simulink subsystem "eulerAngles2Quat"  (R2026a)
settings: Solver=VariableStepAuto
values from neighbouring files (symbols this model uses):
  navControl = 1    [navParams.sldd]
libraries: aerolibutil x1, sharedutil x1
settings Model: Creator=maxhu  LastModifiedBy=maxhu

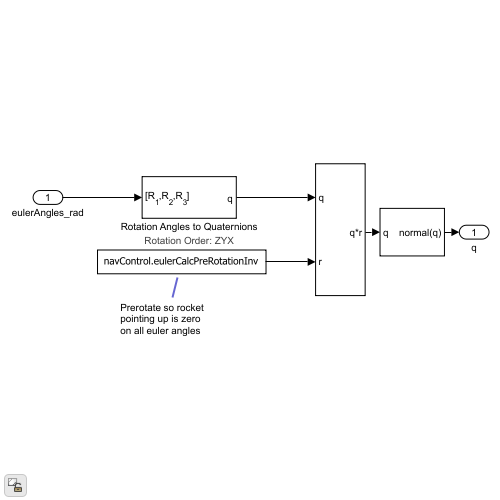
[thumbnail: Simulink's stored preview of the top-level diagram]
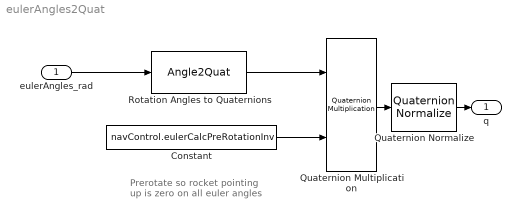
== system eulerAngles2Quat ==
  note: Prerotate so rocket pointing up is zero on all euler angles
  eulerAngles_rad : Inport
  Constant : Constant  Value=navControl.eulerCalcPreRotationInv
  Quaternion Multiplication : aerolibutil/Quaternion Multiplication
  Quaternion Normalize : sharedutil/Quaternion Normalize  aMode=aMode
  Rotation Angles to Quaternions : Angle2Quat
      settings: AttributesFormatString=Rotation Order: %<rotationOrder>
  q : Outport
  wires:
  Constant/1 -> Quaternion Multiplication/2
  eulerAngles_rad/1 -> Rotation Angles to Quaternions/1
  Rotation Angles to Quaternions/1 -> Quaternion Multiplication/1
  Quaternion Normalize/1 -> q/1
  Quaternion Multiplication/1 -> Quaternion Normalize/1
